simulink model "model_2"  (R2021b)
settings: Solver=VariableStepAuto  StartTime=0.0  StopTime=10  RelTol=1e-3
values from neighbouring files (symbols this model uses):
  A = [-5, 0; 0, -10]    [task_1.m]    (also in task_3.m = [0,1;0,0]; task_4.m = [0,1;0,0]; task_5.m = [0,1;0,0]; task_6.m = [0,1;0,0])
  B = [1; 1]    [task_1.m]
  C = [1, -1; 1, 1]    [task_1.m]
undefined symbols (not defined in the file or in its folder): x1, x2, x3, x4
libraries: matrix_library x4
settings Model: Creator=vital  LastModifiedBy=vital

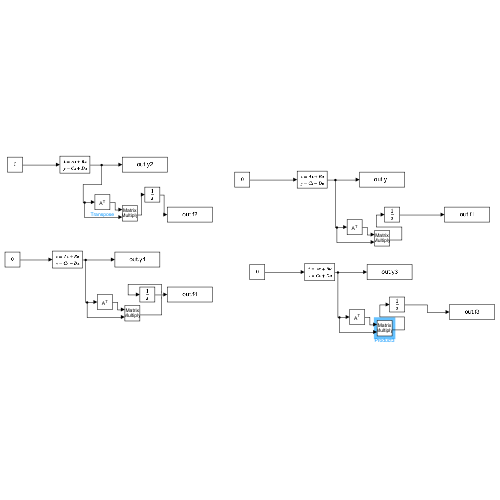
[thumbnail: Simulink's stored preview of the top-level diagram]
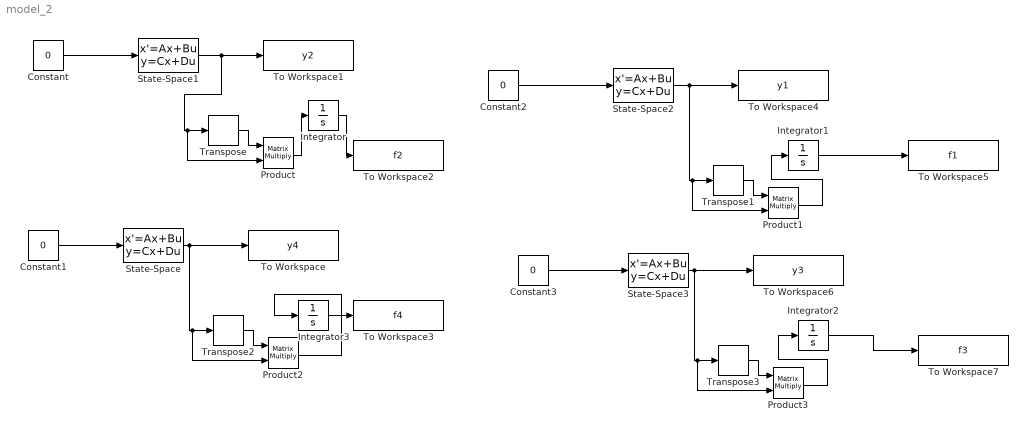
== system model_2 ==
  Constant{,1..3} (4 alike) : Constant  Value=0
  Integrator{,1..3} (4 alike) : Integrator
  Product{,1..3} (4 alike) : Product  Multiplication=Matrix(*)
  State-Space : StateSpace  A=A  B=B  C=C  D=[0; 0]  InitialCondition=x4  ParameterTunability=Optimized
  State-Space1 : StateSpace  A=A  B=B  C=C  D=[0; 0]  InitialCondition=x2
  State-Space2 : StateSpace  A=A  B=B  C=C  D=[0; 0]  InitialCondition=x1
  State-Space3 : StateSpace  A=A  B=B  C=C  D=[0; 0]  InitialCondition=x3  ParameterTunability=Unconstrained
  To Workspace : ToWorkspace  VariableName=y4  SaveFormat=Timeseries  SampleTime=0.0005
  To Workspace1 : ToWorkspace  VariableName=y2  SaveFormat=Timeseries  SampleTime=0.0005
  To Workspace2 : ToWorkspace  VariableName=f2  SaveFormat=Timeseries  SampleTime=0.0005
  To Workspace3 : ToWorkspace  VariableName=f4  SaveFormat=Timeseries  SampleTime=0.0005
  To Workspace4 : ToWorkspace  VariableName=y1  SaveFormat=Timeseries  SampleTime=0.0005
  To Workspace5 : ToWorkspace  VariableName=f1  SaveFormat=Timeseries  SampleTime=0.0005
  To Workspace6 : ToWorkspace  VariableName=y3  SaveFormat=Timeseries  SampleTime=0.0005
  To Workspace7 : ToWorkspace  VariableName=f3  SaveFormat=Timeseries  SampleTime=0.0005
  Transpose{,1..3} (4 alike) : matrix_library/Transpose
      settings: SourceProductBaseCode=SL
  wires:
  State-Space1/1 -> Product/2, Transpose/1, To Workspace1/1
  Constant/1 -> State-Space1/1
  Constant1/1 -> State-Space/1
  Constant2/1 -> State-Space2/1
  Constant3/1 -> State-Space3/1
  Product/1 -> Integrator/1
  Integrator/1 -> To Workspace2/1
  Product1/1 -> Integrator1/1
  Integrator3/1 -> To Workspace3/1
  Product2/1 -> Integrator3/1
  Transpose/1 -> Product/1
  Transpose1/1 -> Product1/1
  State-Space2/1 -> To Workspace4/1, Product1/2, Transpose1/1
  Transpose2/1 -> Product2/1
  State-Space/1 -> To Workspace/1, Product2/2, Transpose2/1
  Transpose3/1 -> Product3/1
  State-Space3/1 -> To Workspace6/1, Product3/2, Transpose3/1
  Product3/1 -> Integrator2/1
  Integrator1/1 -> To Workspace5/1
  Integrator2/1 -> To Workspace7/1
